simulink model "NInvState"  (R2024b)
settings: Solver=FixedStepDiscrete  StartTime=0.0  StopTime=1  FixedStep=0.001  RelTol=1e-3  EnableMultiTasking=on
settings Model: DataDictionary=Master_Dictionary.sldd  EnableAccessToBaseWorkspace=off  Creator=torni  LastModifiedBy=oxbro
settings SolverCC: AlgebraicLoopSolver=TrustRegion
settings DataIOCC: ReturnWorkspaceOutputs=off
settings OptimizationCC: DefaultParameterBehavior=Inlined  EnhancedBackFolding=on  PassReuseOutputArgsAs=Individual arguments  ZeroExternalMemoryAtStartup=off  ZeroInternalMemoryAtStartup=off  MaxStackSize=512  OptimizeBlockOrder=speed  DifferentSizesBufferReuse=on  OptimizationCustomize=off  EfficientTunableParamExpr=on
settings DebuggingCC: ParameterTunabilityLossMsg=error  UnconnectedInputMsg=warning  UnconnectedOutputMsg=warning  UnconnectedLineMsg=warning  ArithmeticOperatorsInVariantConditions=warning
settings HardwareCC: ProdBitPerPointer=32  ProdBitPerSizeT=32  ProdBitPerPtrDiffT=32  ProdLargestAtomicInteger=Long  ProdLargestAtomicFloat=Double  ProdWordSize=32  ProdLongLongMode=on  ProdHWDeviceType=ARM Compatible->ARM Cortex-M
settings ModelReferenceCC: EnableRefExpFcnMdlSchedulingChecks=on
settings SFSimCC: MATLABDynamicMemAlloc=off  CustomCodeUndefinedFunction=UseInterfaceOnly
settings RTWCC: Description=Embedded Coder  SystemTargetFile=ert.tlc  HardwareBoard=STM32H7xx Based (Single-core)  TemplateMakefile=ert_default_tmf  CustomHeaderCode="#include \"stm32h7xx_ll_tim.h\""  CustomInitializer=LL_TIM_EnableCounter(TIM2);  Toolchain=GNU Tools for ARM Embedded Processors  GPUComputeCapability=3.5
settings CodeAppCC: ForceParamTrailComments=on  IgnoreCustomStorageClasses=off  OperatorAnnotations=on  SimulinkDataObjDesc=on  SFDataObjDesc=on  InsertBlockDesc=on
settings ERTTargetCC: TargetLangStandard=C99 (ISO)  CodeReplacementLibrary=ARM Cortex-M  ExtModeTransport=3  ExtModeStaticAlloc=on  ExtModeStaticAllocSize=2048  ExtModeMexFile=ext_xcp  ExtModeIntrfLevel=Level2 - Open

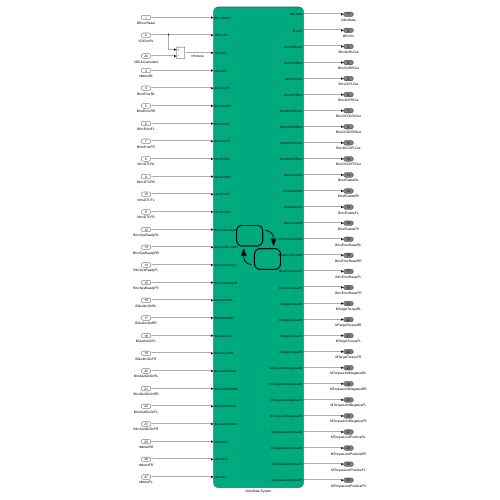
[thumbnail: Simulink's stored preview of the top-level diagram]
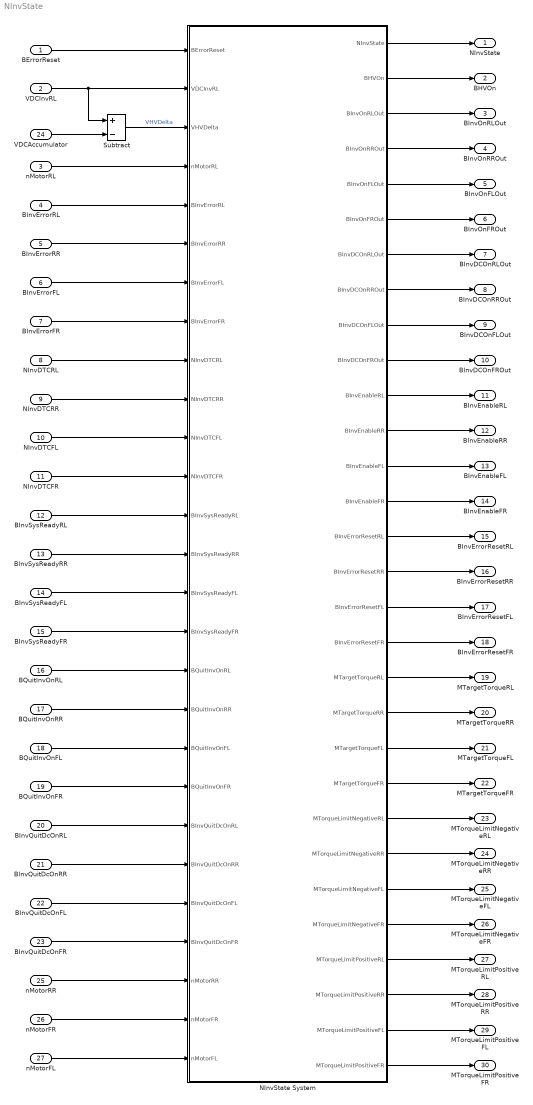
== system NInvState ==
  BErrorReset : Inport  OutDataTypeStr=boolean
  VDCInvRL : Inport  Port=2  OutDataTypeStr=double
  nMotorRL : Inport  Port=3  OutDataTypeStr=double
  BInvErrorRL : Inport  Port=4  OutDataTypeStr=boolean
  BInvErrorRR : Inport  Port=5  OutDataTypeStr=boolean
  BInvErrorFL : Inport  Port=6  OutDataTypeStr=boolean
  BInvErrorFR : Inport  Port=7  OutDataTypeStr=boolean
  NInvDTCRL : Inport  Port=8  OutDataTypeStr=double
  "NInvDTCRR " : Inport  Port=9  OutDataTypeStr=double
  NInvDTCFL : Inport  Port=10  OutDataTypeStr=double
  NInvDTCFR : Inport  Port=11  OutDataTypeStr=double
  BInvSysReadyRL : Inport  Port=12  OutDataTypeStr=boolean
  BInvSysReadyRR : Inport  Port=13  OutDataTypeStr=boolean
  BInvSysReadyFL : Inport  Port=14  OutDataTypeStr=boolean
  BInvSysReadyFR : Inport  Port=15  OutDataTypeStr=boolean
  BQuitInvOnRL : Inport  Port=16  OutDataTypeStr=boolean
  BQuitInvOnRR : Inport  Port=17  OutDataTypeStr=boolean
  BQuitInvOnFL : Inport  Port=18  OutDataTypeStr=boolean
  BQuitInvOnFR : Inport  Port=19  OutDataTypeStr=boolean
  BInvQuitDcOnRL : Inport  Port=20  OutDataTypeStr=boolean
  BInvQuitDcOnRR : Inport  Port=21  OutDataTypeStr=boolean
  BInvQuitDcOnFL : Inport  Port=22  OutDataTypeStr=boolean
  BInvQuitDcOnFR : Inport  Port=23  OutDataTypeStr=boolean
  VDCAccumulator : Inport  Port=24  OutDataTypeStr=double
  nMotorRR : Inport  Port=25  OutDataTypeStr=double
  nMotorFR : Inport  Port=26  OutDataTypeStr=double
  nMotorFL : Inport  Port=27  OutDataTypeStr=double
  NInvState System : Stateflow chart  TreatAsAtomicUnit=on
  Subtract : Sum  Inputs=+-
  NInvState : Outport  OutDataTypeStr=double  VectorParamsAs1DForOutWhenUnconnected=off
  BHVOn : Outport  Port=2  OutDataTypeStr=double  VectorParamsAs1DForOutWhenUnconnected=off
  BInvOnRLOut : Outport  Port=3  OutDataTypeStr=double  VectorParamsAs1DForOutWhenUnconnected=off
  BInvOnRROut : Outport  Port=4  OutDataTypeStr=double  VectorParamsAs1DForOutWhenUnconnected=off
  BInvOnFLOut : Outport  Port=5  OutDataTypeStr=double  VectorParamsAs1DForOutWhenUnconnected=off
  BInvOnFROut : Outport  Port=6  OutDataTypeStr=double  VectorParamsAs1DForOutWhenUnconnected=off
  BInvDCOnRLOut : Outport  Port=7  OutDataTypeStr=double  VectorParamsAs1DForOutWhenUnconnected=off
  BInvDCOnRROut : Outport  Port=8  OutDataTypeStr=double  VectorParamsAs1DForOutWhenUnconnected=off
  BInvDCOnFLOut : Outport  Port=9  OutDataTypeStr=double  VectorParamsAs1DForOutWhenUnconnected=off
  BInvDCOnFROut : Outport  Port=10  OutDataTypeStr=double  VectorParamsAs1DForOutWhenUnconnected=off
  BInvEnableRL : Outport  Port=11  OutDataTypeStr=double  VectorParamsAs1DForOutWhenUnconnected=off
  BInvEnableRR : Outport  Port=12  OutDataTypeStr=double  VectorParamsAs1DForOutWhenUnconnected=off
  BInvEnableFL : Outport  Port=13  OutDataTypeStr=double  VectorParamsAs1DForOutWhenUnconnected=off
  BInvEnableFR : Outport  Port=14  OutDataTypeStr=double  VectorParamsAs1DForOutWhenUnconnected=off
  BInvErrorResetRL : Outport  Port=15  OutDataTypeStr=double  VectorParamsAs1DForOutWhenUnconnected=off
  BInvErrorResetRR : Outport  Port=16  OutDataTypeStr=double  VectorParamsAs1DForOutWhenUnconnected=off
  BInvErrorResetFL : Outport  Port=17  OutDataTypeStr=double  VectorParamsAs1DForOutWhenUnconnected=off
  BInvErrorResetFR : Outport  Port=18  OutDataTypeStr=double  VectorParamsAs1DForOutWhenUnconnected=off
  MTargetTorqueRL : Outport  Port=19  OutDataTypeStr=double  VectorParamsAs1DForOutWhenUnconnected=off
  MTargetTorqueRR : Outport  Port=20  OutDataTypeStr=double  VectorParamsAs1DForOutWhenUnconnected=off
  MTargetTorqueFL : Outport  Port=21  OutDataTypeStr=double  VectorParamsAs1DForOutWhenUnconnected=off
  MTargetTorqueFR : Outport  Port=22  OutDataTypeStr=double  VectorParamsAs1DForOutWhenUnconnected=off
  MTorqueLimitNegativeRL : Outport  Port=23  OutDataTypeStr=double  VectorParamsAs1DForOutWhenUnconnected=off
  MTorqueLimitNegativeRR : Outport  Port=24  OutDataTypeStr=double  VectorParamsAs1DForOutWhenUnconnected=off
  MTorqueLimitNegativeFL : Outport  Port=25  OutDataTypeStr=double  VectorParamsAs1DForOutWhenUnconnected=off
  MTorqueLimitNegativeFR : Outport  Port=26  OutDataTypeStr=double  VectorParamsAs1DForOutWhenUnconnected=off
  MTorqueLimitPositiveRL : Outport  Port=27  OutDataTypeStr=double  VectorParamsAs1DForOutWhenUnconnected=off
  MTorqueLimitPositiveRR : Outport  Port=28  OutDataTypeStr=double  VectorParamsAs1DForOutWhenUnconnected=off
  MTorqueLimitPositiveFL : Outport  Port=29  OutDataTypeStr=double  VectorParamsAs1DForOutWhenUnconnected=off
  MTorqueLimitPositiveFR : Outport  Port=30  OutDataTypeStr=double  VectorParamsAs1DForOutWhenUnconnected=off
  wires:
  BErrorReset/1 -> NInvState System/1(BErrorReset)
  VDCInvRL/1 -> Subtract/1, NInvState System/2(VDCInvRL)
  nMotorRL/1 -> NInvState System/4(nMotorRL)
  BInvErrorRL/1 -> NInvState System/5(BInvErrorRL)
  BInvErrorRR/1 -> NInvState System/6(BInvErrorRR)
  BInvErrorFL/1 -> NInvState System/7(BInvErrorFL)
  BInvErrorFR/1 -> NInvState System/8(BInvErrorFR)
  NInvDTCRL/1 -> NInvState System/9(NInvDTCRL)
  "NInvDTCRR "/1 -> NInvState System/10(NInvDTCRR)
  NInvDTCFL/1 -> NInvState System/11(NInvDTCFL)
  NInvDTCFR/1 -> NInvState System/12(NInvDTCFR)
  BInvSysReadyRL/1 -> NInvState System/13(BInvSysReadyRL)
  BInvSysReadyRR/1 -> NInvState System/14(BInvSysReadyRR)
  BInvSysReadyFL/1 -> NInvState System/15(BInvSysReadyFL)
  BInvSysReadyFR/1 -> NInvState System/16(BInvSysReadyFR)
  BQuitInvOnRL/1 -> NInvState System/17(BQuitInvOnRL)
  BQuitInvOnRR/1 -> NInvState System/18(BQuitInvOnRR)
  BQuitInvOnFL/1 -> NInvState System/19(BQuitInvOnFL)
  BQuitInvOnFR/1 -> NInvState System/20(BQuitInvOnFR)
  BInvQuitDcOnRL/1 -> NInvState System/21(BInvQuitDcOnRL)
  BInvQuitDcOnFL/1 -> NInvState System/23(BInvQuitDcOnFL)
  BInvQuitDcOnRR/1 -> NInvState System/22(BInvQuitDcOnRR)
  BInvQuitDcOnFR/1 -> NInvState System/24(BInvQuitDcOnFR)
  VDCAccumulator/1 -> Subtract/2
  Subtract/1 -> NInvState System/3(VHVDelta)  "VHVDelta"
  NInvState System/2(BHVOn) -> BHVOn/1
  NInvState System/1(NInvState) -> NInvState/1
  NInvState System/3(BInvOnRLOut) -> BInvOnRLOut/1
  NInvState System/4(BInvOnRROut) -> BInvOnRROut/1
  NInvState System/5(BInvOnFLOut) -> BInvOnFLOut/1
  NInvState System/6(BInvOnFROut) -> BInvOnFROut/1
  NInvState System/7(BInvDCOnRLOut) -> BInvDCOnRLOut/1
  NInvState System/8(BInvDCOnRROut) -> BInvDCOnRROut/1
  NInvState System/9(BInvDCOnFLOut) -> BInvDCOnFLOut/1
  NInvState System/10(BInvDCOnFROut) -> BInvDCOnFROut/1
  NInvState System/11(BInvEnableRL) -> BInvEnableRL/1
  NInvState System/12(BInvEnableRR) -> BInvEnableRR/1
  NInvState System/13(BInvEnableFL) -> BInvEnableFL/1
  NInvState System/14(BInvEnableFR) -> BInvEnableFR/1
  NInvState System/15(BInvErrorResetRL) -> BInvErrorResetRL/1
  NInvState System/16(BInvErrorResetRR) -> BInvErrorResetRR/1
  NInvState System/17(BInvErrorResetFL) -> BInvErrorResetFL/1
  NInvState System/18(BInvErrorResetFR) -> BInvErrorResetFR/1
  NInvState System/19(MTargetTorqueRL) -> MTargetTorqueRL/1
  NInvState System/20(MTargetTorqueRR) -> MTargetTorqueRR/1
  NInvState System/21(MTargetTorqueFL) -> MTargetTorqueFL/1
  NInvState System/22(MTargetTorqueFR) -> MTargetTorqueFR/1
  NInvState System/23(MTorqueLimitNegativeRL) -> MTorqueLimitNegativeRL/1
  NInvState System/24(MTorqueLimitNegativeRR) -> MTorqueLimitNegativeRR/1
  NInvState System/25(MTorqueLimitNegativeFL) -> MTorqueLimitNegativeFL/1
  NInvState System/26(MTorqueLimitNegativeFR) -> MTorqueLimitNegativeFR/1
  NInvState System/27(MTorqueLimitPositiveRL) -> MTorqueLimitPositiveRL/1
  NInvState System/28(MTorqueLimitPositiveRR) -> MTorqueLimitPositiveRR/1
  NInvState System/29(MTorqueLimitPositiveFL) -> MTorqueLimitPositiveFL/1
  NInvState System/30(MTorqueLimitPositiveFR) -> MTorqueLimitPositiveFR/1
  nMotorRR/1 -> NInvState System/25(nMotorRR)
  nMotorFR/1 -> NInvState System/26(nMotorFR)
  nMotorFL/1 -> NInvState System/27(nMotorFL)

== stateflow chart NInvState/NInvState System ==
  state Inv_State_Idle
    entry:
    NInvState=0;
  state Inverter_DCOFF
    entry:
    BInvDCOnFLOut = 0
    BInvDCOnFROut = 0
    BInvDCOnRLOut = 0
    BInvDCOnRROut = 0
  state Inv_Error_Checks
    state Inv_LV_Check2
      entry:
      NInvState=2
      BInvErrorResetRR=0;
      BInvErrorResetRL=0;
      BInvErrorResetFR=0;
      BInvErrorResetFL=0;
    state Inv_LV_Check1
      entry:
      BInvErrorResetRR=1;
      BInvErrorResetRL=1;
      BInvErrorResetFR=1;
      BInvErrorResetFL=1;
    state Inv_LV_OK
      entry:
      NInvState=3;
    state Inv_LV_Check
      entry:
      NInvState=1;
      BInvErrorResetRR=0;
      BInvErrorResetRL=0;
      BInvErrorResetFR=0;
      BInvErrorResetFL=0;
    Inv_LV_Check1 -> Inv_LV_Check2 : after(100, tick)
        | [BInvErrorFL==0&&...
        | BInvErrorFR==0&&...
        | BInvErrorRR==0&&...
        | BInvErrorRL==0]
    (default) -> Inv_LV_Check
    Inv_LV_Check2 -> Inv_LV_Check [order 1] : [BInvErrorRR==1 ||...
        | BInvErrorRL==1 ||...
        | BInvErrorFR==1 ||...
        | BInvErrorFL==1]
    Inv_LV_Check2 -> Inv_LV_OK [order 2] : [BInvErrorRR==0 &&...
        | BInvErrorRL==0 &&...
        | BInvErrorFR==0 &&...
        | BInvErrorFL==0 &&...
        | BInvSysReadyRL==1 &&...
        | BInvSysReadyRR==1 &&...
        | BInvSysReadyFL==1 &&...
        | BInvSysReadyFR==1]
    Inv_LV_Check -> Inv_LV_Check1 : after(100,tick)
    Inv_LV_OK -> Inv_LV_Check : [BErrorReset==1 && nMotorRL<500]
  state Inv_OK
    entry:
    NInvState=92
  state Encoder_Reset_RL
    state Encoder_Error_RL
      entry:
      NInvState=404
      state PBX_SENSORS_ini
        entry:
        BInvErrorResetRL=0;
      state Error_On
        entry:
        BInvErrorResetRL=1;
      state Error_off
        entry:
        BInvErrorResetRL=0;
      (default) -> Encoder_Reset_RL.Encoder_Error_RL.PBX_SENSORS_ini
      Encoder_Reset_RL.Encoder_Error_RL.PBX_SENSORS_ini -> Encoder_Reset_RL.Encoder_Error_RL.Error_On : after(50, tick)
      Encoder_Reset_RL.Encoder_Error_RL.Error_off -> Encoder_Reset_RL.Encoder_Error_RL.PBX_SENSORS_ini [order 2] : [BInvErrorRL ==1]
      Encoder_Reset_RL.Encoder_Error_RL.Error_On -> Encoder_Reset_RL.Encoder_Error_RL.Error_off : after(100, tick)
          | [BInvErrorRL ==0]
    state Inverter_HV_Checks3
      exit:
      BHVOn=1
      state Inverter_IN
        entry:
        NInvState = 22
        BInvDCOnRLOut = 1
      state Inv_Error_Check_2
        BInvErrorResetRL = 0
      state Inv_Error_Reset
        entry:
        BInvErrorResetRL=1
        BInvDCOnRLOut=0
        BInvEnableRL = 0
        BInvOnRLOut = 0
      state START_UP
        entry:
        NInvState = 23
        MTargetTorqueRL=0
        MTorqueLimitNegativeRL = 0
        MTorqueLimitPositiveRL = 0
        BInvEnableRL = 1
      state Inv_Error_Check_1
        entry:
        NInvState = 00
        MTorqueLimitNegativeRL = 0
        MTorqueLimitPositiveRL = 0
      state Inverter_ON
        entry:
        NInvState = 24
        BInvOnRLOut = 1
      state TorqueReq_Ready
        entry:
        NInvState = 25
        MTorqueLimitNegativeRL = -204.1
        MTorqueLimitPositiveRL = 214.2
      (default) -> Encoder_Reset_RL.Inverter_HV_Checks3.Inverter_IN
      (junction 784) -> Encoder_Reset_RL.Inverter_HV_Checks3.Inverter_IN [order 1] : [BInvErrorRL==0]
      Encoder_Reset_RL.Inverter_HV_Checks3.Inv_Error_Check_2 -> (junction 784) : after(500,tick)
      (junction 784) -> Encoder_Reset_RL.Inverter_HV_Checks3.Inv_Error_Check_1 [order 2] : [BInvErrorRL==1]
      Encoder_Reset_RL.Inverter_HV_Checks3.Inv_Error_Reset -> Encoder_Reset_RL.Inverter_HV_Checks3.Inv_Error_Check_2 : after(500,tick)
      Encoder_Reset_RL.Inverter_HV_Checks3.Inverter_IN -> Encoder_Reset_RL.Inverter_HV_Checks3.START_UP : [BInvQuitDcOnRL==1]
      Encoder_Reset_RL.Inverter_HV_Checks3.START_UP -> Encoder_Reset_RL.Inverter_HV_Checks3.Inverter_ON : after(100,tick)
      Encoder_Reset_RL.Inverter_HV_Checks3.Inv_Error_Check_1 -> Encoder_Reset_RL.Inverter_HV_Checks3.Inv_Error_Reset : after(500,tick)
      Encoder_Reset_RL.Inverter_HV_Checks3.Inverter_ON -> Encoder_Reset_RL.Inverter_HV_Checks3.TorqueReq_Ready [order 1] : [BQuitInvOnRL == 1]
      Encoder_Reset_RL.Inverter_HV_Checks3.Inverter_ON -> Encoder_Reset_RL.Inverter_HV_Checks3.Inv_Error_Check_1 [order 2] : [BInvErrorRL==1]
      Encoder_Reset_RL.Inverter_HV_Checks3.TorqueReq_Ready -> Encoder_Reset_RL.Inverter_HV_Checks3.Inv_Error_Check_1 [order 1] : [BInvErrorRL==1]
    state Encoder_OK
      entry:
      NInvState = 26
    (default) -> Encoder_Error_RL
    Encoder_Reset_RL.Encoder_Error_RL.Error_off -> Encoder_Reset_RL.Inverter_HV_Checks3 [order 1] : [BInvSysReadyRL==1]
    Encoder_Reset_RL.Inverter_HV_Checks3.TorqueReq_Ready -> Encoder_Reset_RL.Encoder_OK [order 2] : [BInvErrorRL==0]
  state Encoder_Reset_RR
    state Encoder_Error_RR
      entry:
      NInvState = 404
      state PBX_SENSORS_ini
        entry:
        BInvErrorResetRR=0;
      state Error_On
        entry:
        BInvErrorResetRR=1;
      state Error_off
        entry:
        BInvErrorResetRR=0;
      (default) -> Encoder_Reset_RR.Encoder_Error_RR.PBX_SENSORS_ini
      Encoder_Reset_RR.Encoder_Error_RR.PBX_SENSORS_ini -> Encoder_Reset_RR.Encoder_Error_RR.Error_On : after(50, tick)
      Encoder_Reset_RR.Encoder_Error_RR.Error_off -> Encoder_Reset_RR.Encoder_Error_RR.PBX_SENSORS_ini [order 2] : [BInvErrorRR ==1]
      Encoder_Reset_RR.Encoder_Error_RR.Error_On -> Encoder_Reset_RR.Encoder_Error_RR.Error_off : after(100, tick)
          | [BInvErrorRR ==0]
    state Inverter_HV_CheckRR
      exit:
      BHVOn=1
      state Inverter_IN
        entry:
        NInvState = 27
        BInvDCOnRROut = 1
      state Inv_Error_Check_2
        BInvErrorResetRR = 0
      state Inv_Error_Reset
        entry:
        BInvErrorResetRR=1
        BInvDCOnRROut=0
        BInvEnableRR = 0
        BInvOnRROut = 0
      state START_UP
        entry:
        NInvState = 28
        MTargetTorqueRR=0
        MTorqueLimitNegativeRR = 0
        MTorqueLimitPositiveRR = 0
        BInvEnableRR = 1
      state Inv_Error_Check_1
        entry:
        MTorqueLimitNegativeRR = 0
        MTorqueLimitPositiveRR = 0
      state Inverter_ON
        entry:
        NInvState = 29
        BInvOnRROut = 1
      state TorqueReq_Ready
        entry:
        NInvState = 30
        MTorqueLimitNegativeRR = -204.1
        MTorqueLimitPositiveRR = 214.2
      (default) -> Encoder_Reset_RR.Inverter_HV_CheckRR.Inverter_IN
      (junction 861) -> Encoder_Reset_RR.Inverter_HV_CheckRR.Inverter_IN [order 1] : [BInvErrorRR==0]
      Encoder_Reset_RR.Inverter_HV_CheckRR.Inv_Error_Check_2 -> (junction 861) : after(500,tick)
      (junction 861) -> Encoder_Reset_RR.Inverter_HV_CheckRR.Inv_Error_Check_1 [order 2] : [BInvErrorRR==1]
      Encoder_Reset_RR.Inverter_HV_CheckRR.Inv_Error_Reset -> Encoder_Reset_RR.Inverter_HV_CheckRR.Inv_Error_Check_2 : after(500,tick)
      Encoder_Reset_RR.Inverter_HV_CheckRR.Inverter_IN -> Encoder_Reset_RR.Inverter_HV_CheckRR.START_UP : [BInvQuitDcOnRR==1]
      Encoder_Reset_RR.Inverter_HV_CheckRR.START_UP -> Encoder_Reset_RR.Inverter_HV_CheckRR.Inverter_ON : after(100,tick)
      Encoder_Reset_RR.Inverter_HV_CheckRR.Inv_Error_Check_1 -> Encoder_Reset_RR.Inverter_HV_CheckRR.Inv_Error_Reset : after(500,tick)
      Encoder_Reset_RR.Inverter_HV_CheckRR.Inverter_ON -> Encoder_Reset_RR.Inverter_HV_CheckRR.TorqueReq_Ready [order 1] : [BQuitInvOnRR == 1]
      Encoder_Reset_RR.Inverter_HV_CheckRR.Inverter_ON -> Encoder_Reset_RR.Inverter_HV_CheckRR.Inv_Error_Check_1 [order 2] : [BInvErrorRR==1]
      Encoder_Reset_RR.Inverter_HV_CheckRR.TorqueReq_Ready -> Encoder_Reset_RR.Inverter_HV_CheckRR.Inv_Error_Check_1 [order 1] : [BInvErrorRR==1]
    state Encoder_OK
      entry:
      NInvState = 31
    (default) -> Encoder_Error_RR
    Encoder_Reset_RR.Encoder_Error_RR.Error_off -> Encoder_Reset_RR.Inverter_HV_CheckRR [order 1] : [BInvSysReadyRR==1]
    Encoder_Reset_RR.Inverter_HV_CheckRR.TorqueReq_Ready -> Encoder_Reset_RR.Encoder_OK [order 2] : [BInvErrorRR==0]
  state Encoder_Reset_FL
    state Encoder_Error_FL
      entry:
      NInvState = 404
      state Error_On
        entry:
        BInvErrorResetFL=1;
      state PBX_SENSORS_ini
        entry:
        BInvErrorResetFL=0;
      state Error_off
        entry:
        BInvErrorResetFL=0;
      (default) -> Encoder_Reset_FL.Encoder_Error_FL.PBX_SENSORS_ini
      Encoder_Reset_FL.Encoder_Error_FL.PBX_SENSORS_ini -> Encoder_Reset_FL.Encoder_Error_FL.Error_On : after(50, tick)
      Encoder_Reset_FL.Encoder_Error_FL.Error_off -> Encoder_Reset_FL.Encoder_Error_FL.PBX_SENSORS_ini [order 2] : [BInvErrorFL ==1]
      Encoder_Reset_FL.Encoder_Error_FL.Error_On -> Encoder_Reset_FL.Encoder_Error_FL.Error_off : after(100, tick)
          | [BInvErrorFL ==0]
    state Inverter_HV_Checks2
      exit:
      BHVOn=1
      state Inverter_IN
        entry:
        NInvState = 32
        BInvDCOnFLOut = 1
      state Inv_Error_Check_2
        BInvErrorResetFL = 0
      state Inv_Error_Reset
        entry:
        BInvErrorResetFL=1
        BInvDCOnFLOut=0
        BInvEnableFL = 0
        BInvOnFLOut = 0
      state START_UP
        entry:
        NInvState = 33
        MTargetTorqueFL=0
        MTorqueLimitNegativeFL = 0
        MTorqueLimitPositiveFL = 0
        BInvEnableFL = 1
      state Inv_Error_Check_1
        entry:
        MTorqueLimitNegativeFL = 0
        MTorqueLimitPositiveFL = 0
      state Inverter_ON
        entry:
        NInvState = 34
        BInvOnFLOut = 1
      state TorqueReq_Ready
        entry:
        NInvState = 35
        MTorqueLimitNegativeFL = -204.1
        MTorqueLimitPositiveFL = 214.2
      (default) -> Encoder_Reset_FL.Inverter_HV_Checks2.Inverter_IN
      (junction 751) -> Encoder_Reset_FL.Inverter_HV_Checks2.Inverter_IN [order 1] : [BInvErrorFL==0]
      Encoder_Reset_FL.Inverter_HV_Checks2.Inv_Error_Check_2 -> (junction 751) : after(500,tick)
      (junction 751) -> Encoder_Reset_FL.Inverter_HV_Checks2.Inv_Error_Check_1 [order 2] : [BInvErrorFL==1]
      Encoder_Reset_FL.Inverter_HV_Checks2.Inv_Error_Reset -> Encoder_Reset_FL.Inverter_HV_Checks2.Inv_Error_Check_2 : after(500,tick)
      Encoder_Reset_FL.Inverter_HV_Checks2.Inverter_IN -> Encoder_Reset_FL.Inverter_HV_Checks2.START_UP : [BInvQuitDcOnFL==1]
      Encoder_Reset_FL.Inverter_HV_Checks2.START_UP -> Encoder_Reset_FL.Inverter_HV_Checks2.Inverter_ON : after(100,tick)
      Encoder_Reset_FL.Inverter_HV_Checks2.Inv_Error_Check_1 -> Encoder_Reset_FL.Inverter_HV_Checks2.Inv_Error_Reset : after(500,tick)
      Encoder_Reset_FL.Inverter_HV_Checks2.Inverter_ON -> Encoder_Reset_FL.Inverter_HV_Checks2.TorqueReq_Ready [order 1] : [BQuitInvOnFL == 1]
      Encoder_Reset_FL.Inverter_HV_Checks2.Inverter_ON -> Encoder_Reset_FL.Inverter_HV_Checks2.Inv_Error_Check_1 [order 2] : [BInvErrorFL==1]
      Encoder_Reset_FL.Inverter_HV_Checks2.TorqueReq_Ready -> Encoder_Reset_FL.Inverter_HV_Checks2.Inv_Error_Check_1 [order 1] : [BInvErrorFL==1]
    state Encoder_OK
      entry:
      NInvState = 36
    (default) -> Encoder_Error_FL
    Encoder_Reset_FL.Encoder_Error_FL.Error_off -> Inverter_HV_Checks2 [order 1] : [BInvSysReadyFL==1]
    Encoder_Reset_FL.Inverter_HV_Checks2.TorqueReq_Ready -> Encoder_Reset_FL.Encoder_OK [order 2] : [BInvErrorFL==0]
  state Inverter_HV_Checks
    state Inverter_HV_CheckFR
      exit:
      BHVOn=1;
      NInvState = 4
      state Inverter_IN
        entry:
        NInvState = 5
        BInvDCOnFROut = 1
      state Inv_Error_Check_2
        BInvErrorResetFR = 0
      state Inv_Error_Reset
        entry:
        BInvErrorResetFR=1
        BInvDCOnFROut=0
        BInvEnableFR = 0
        BInvOnFROut = 0
      state START_UP
        entry:
        NInvState = 6
        MTargetTorqueFR=0
        MTorqueLimitNegativeFR = 0
        MTorqueLimitPositiveFR = 0
        BInvEnableFR = 1
      state Inv_Error_Check_1
        entry:
        MTorqueLimitNegativeFR = 0
        MTorqueLimitPositiveFR = 0
      state Inverter_ON
        entry:
        NInvState = 7
        BInvOnFROut = 1
      state TorqueReq_Ready
        entry:
        NInvState = 8
        MTorqueLimitNegativeFR = -204.1
        MTorqueLimitPositiveFR = 214.2
      (default) -> Inverter_HV_Checks.Inverter_HV_CheckFR.Inverter_IN
      (junction 1179) -> Inverter_HV_Checks.Inverter_HV_CheckFR.Inverter_IN [order 1] : [BInvErrorFR==0]
      Inverter_HV_Checks.Inverter_HV_CheckFR.Inv_Error_Check_2 -> (junction 1179) : after(500,tick)
      (junction 1179) -> Inverter_HV_Checks.Inverter_HV_CheckFR.Inv_Error_Check_1 [order 2] : [BInvErrorFR==1]
      Inverter_HV_Checks.Inverter_HV_CheckFR.Inverter_IN -> Inverter_HV_Checks.Inverter_HV_CheckFR.Inv_Error_Reset [order 2] : after(500,tick)[BInvErrorFR==1]
      Inverter_HV_Checks.Inverter_HV_CheckFR.Inv_Error_Reset -> Inverter_HV_Checks.Inverter_HV_CheckFR.Inv_Error_Check_2 : after(500,tick)
      Inverter_HV_Checks.Inverter_HV_CheckFR.Inverter_IN -> Inverter_HV_Checks.Inverter_HV_CheckFR.START_UP [order 1] : [BInvQuitDcOnFR==1]
      Inverter_HV_Checks.Inverter_HV_CheckFR.START_UP -> Inverter_HV_Checks.Inverter_HV_CheckFR.Inverter_ON : after(100,tick)
      Inverter_HV_Checks.Inverter_HV_CheckFR.Inv_Error_Check_1 -> Inverter_HV_Checks.Inverter_HV_CheckFR.Inv_Error_Reset : after(500,tick)
      Inverter_HV_Checks.Inverter_HV_CheckFR.Inverter_ON -> Inverter_HV_Checks.Inverter_HV_CheckFR.TorqueReq_Ready [order 1] : [BQuitInvOnFR == 1]
      Inverter_HV_Checks.Inverter_HV_CheckFR.Inverter_ON -> Inverter_HV_Checks.Inverter_HV_CheckFR.Inv_Error_Check_1 [order 2] : [BInvErrorFR==1]
      Inverter_HV_Checks.Inverter_HV_CheckFR.TorqueReq_Ready -> Inverter_HV_Checks.Inverter_HV_CheckFR.Inv_Error_Check_1 [order 2] : [BInvErrorFR==1]
    state Inv_HV_Check
    note: FRONT RIGHT INVERTER
    state Inverter_HV_CheckRR
      exit:
      BHVOn=1
      state Inverter_IN
        entry:
        NInvState = 9;
        BInvDCOnRROut = 1
      state Inv_Error_Check_2
        BInvErrorResetRR = 0
      state Inv_Error_Reset
        entry:
        BInvErrorResetRR=1
        BInvDCOnRROut=0
        BInvEnableRR = 0
        BInvOnRROut = 0
      state START_UP
        entry:
        NInvState = 10
        MTargetTorqueRR=0
        MTorqueLimitNegativeRR = 0
        MTorqueLimitPositiveRR = 0
        BInvEnableRR = 1
      state Inv_Error_Check_1
        entry:
        MTorqueLimitNegativeRR = 0
        MTorqueLimitPositiveRR = 0
      state Inverter_ON
        entry:
        NInvState = 11
        BInvOnRROut = 1
      state TorqueReq_Ready
        entry:
        NInvState = 12
        MTorqueLimitNegativeRR = -204.1
        MTorqueLimitPositiveRR = 214.2
      (default) -> Inverter_HV_Checks.Inverter_HV_CheckRR.Inverter_IN
      (junction 1201) -> Inverter_HV_Checks.Inverter_HV_CheckRR.Inverter_IN [order 1] : [BInvErrorRR==0]
      Inverter_HV_Checks.Inverter_HV_CheckRR.Inv_Error_Check_2 -> (junction 1201) : after(500,tick)
      (junction 1201) -> Inverter_HV_Checks.Inverter_HV_CheckRR.Inv_Error_Check_1 [order 2] : [BInvErrorRR==1]
      Inverter_HV_Checks.Inverter_HV_CheckRR.Inverter_IN -> Inverter_HV_Checks.Inverter_HV_CheckRR.Inv_Error_Reset [order 2] : after(500,tick)[BInvErrorRR==1]
      Inverter_HV_Checks.Inverter_HV_CheckRR.Inv_Error_Reset -> Inverter_HV_Checks.Inverter_HV_CheckRR.Inv_Error_Check_2 : after(500,tick)
      Inverter_HV_Checks.Inverter_HV_CheckRR.Inverter_IN -> Inverter_HV_Checks.Inverter_HV_CheckRR.START_UP [order 1] : [BInvQuitDcOnRR==1]
      Inverter_HV_Checks.Inverter_HV_CheckRR.START_UP -> Inverter_HV_Checks.Inverter_HV_CheckRR.Inverter_ON : after(100,tick)
      Inverter_HV_Checks.Inverter_HV_CheckRR.Inv_Error_Check_1 -> Inverter_HV_Checks.Inverter_HV_CheckRR.Inv_Error_Reset : after(500,tick)
      Inverter_HV_Checks.Inverter_HV_CheckRR.Inverter_ON -> Inverter_HV_Checks.Inverter_HV_CheckRR.TorqueReq_Ready [order 1] : [BQuitInvOnRR == 1]
      Inverter_HV_Checks.Inverter_HV_CheckRR.Inverter_ON -> Inverter_HV_Checks.Inverter_HV_CheckRR.Inv_Error_Check_1 [order 2] : [BInvErrorRR==1]
      Inverter_HV_Checks.Inverter_HV_CheckRR.TorqueReq_Ready -> Inverter_HV_Checks.Inverter_HV_CheckRR.Inv_Error_Check_1 [order 2] : [BInvErrorRR==1]
    note: REAR RIGHT INVERTER
    state Inverter_HV_ChecksFL
      exit:
      BHVOn=1
      state Inverter_IN
        entry:
        NInvState = 13
        BInvDCOnFLOut = 1
      state Inv_Error_Check_2
        BInvErrorResetFL = 0
      state Inv_Error_Reset
        entry:
        BInvErrorResetFL=1
        BInvDCOnFLOut=0
        BInvEnableFL = 0
        BInvOnFLOut = 0
      state START_UP
        entry:
        NInvState = 14
        MTargetTorqueFL=0
        MTorqueLimitNegativeFL = 0
        MTorqueLimitPositiveFL = 0
        BInvEnableFL = 1
      state Inv_Error_Check_1
        entry:
        MTorqueLimitNegativeFL = 0
        MTorqueLimitPositiveFL = 0
      state Inverter_ON
        entry:
        NInvState = 15
        BInvOnFLOut = 1
      state TorqueReq_Ready
        entry:
        NInvState = 16
        MTorqueLimitNegativeFL = -204.1
        MTorqueLimitPositiveFL = 214.2
      (default) -> Inverter_HV_Checks.Inverter_HV_ChecksFL.Inverter_IN
      (junction 1222) -> Inverter_HV_Checks.Inverter_HV_ChecksFL.Inverter_IN [order 1] : [BInvErrorFL==0]
      Inverter_HV_Checks.Inverter_HV_ChecksFL.Inv_Error_Check_2 -> (junction 1222) : after(500,tick)
      (junction 1222) -> Inverter_HV_Checks.Inverter_HV_ChecksFL.Inv_Error_Check_1 [order 2] : [BInvErrorFL==1]
      Inverter_HV_Checks.Inverter_HV_ChecksFL.Inverter_IN -> Inverter_HV_Checks.Inverter_HV_ChecksFL.Inv_Error_Reset [order 2] : after(500,tick)[BInvErrorFL==1]
      Inverter_HV_Checks.Inverter_HV_ChecksFL.Inv_Error_Reset -> Inverter_HV_Checks.Inverter_HV_ChecksFL.Inv_Error_Check_2 : after(500,tick)
      Inverter_HV_Checks.Inverter_HV_ChecksFL.Inverter_IN -> Inverter_HV_Checks.Inverter_HV_ChecksFL.START_UP [order 1] : [BInvQuitDcOnFL==1]
      Inverter_HV_Checks.Inverter_HV_ChecksFL.START_UP -> Inverter_HV_Checks.Inverter_HV_ChecksFL.Inverter_ON : after(100,tick)
      Inverter_HV_Checks.Inverter_HV_ChecksFL.Inv_Error_Check_1 -> Inverter_HV_Checks.Inverter_HV_ChecksFL.Inv_Error_Reset : after(500,tick)
      Inverter_HV_Checks.Inverter_HV_ChecksFL.Inverter_ON -> Inverter_HV_Checks.Inverter_HV_ChecksFL.TorqueReq_Ready [order 1] : [BQuitInvOnFL == 1]
      Inverter_HV_Checks.Inverter_HV_ChecksFL.Inverter_ON -> Inverter_HV_Checks.Inverter_HV_ChecksFL.Inv_Error_Check_1 [order 2] : [BInvErrorFL==1]
      Inverter_HV_Checks.Inverter_HV_ChecksFL.TorqueReq_Ready -> Inverter_HV_Checks.Inverter_HV_ChecksFL.Inv_Error_Check_1 [order 2] : [BInvErrorFL==1]
    note: FRONT LEFT INVERTER
    state Inverter_HV_ChecksRL
      exit:
      BHVOn=1
      state Inverter_IN
        entry:
        NInvState = 17
        BInvDCOnRLOut = 1
      state Inv_Error_Check_2
        BInvErrorResetRL = 0
      state Inv_Error_Reset
        entry:
        BInvErrorResetRL=1
        BInvDCOnRLOut=0
        BInvEnableRL = 0
        BInvOnRLOut = 0
      state START_UP
        entry:
        NInvState = 18
        MTargetTorqueRL=0
        MTorqueLimitNegativeRL = 0
        MTorqueLimitPositiveRL = 0
        BInvEnableRL = 1
      state Inv_Error_Check_1
        entry:
        MTorqueLimitNegativeRL = 0
        MTorqueLimitPositiveRL = 0
      state Inverter_ON
        entry:
        NInvState = 19
        BInvOnRLOut = 1
      state TorqueReq_Ready
        entry:
        NInvState = 20
        MTorqueLimitNegativeRL = -204.1
        MTorqueLimitPositiveRL = 214.2
      (default) -> Inverter_HV_Checks.Inverter_HV_ChecksRL.Inverter_IN
      (junction 1243) -> Inverter_HV_Checks.Inverter_HV_ChecksRL.Inverter_IN [order 1] : [BInvErrorRL==0]
      Inverter_HV_Checks.Inverter_HV_ChecksRL.Inv_Error_Check_2 -> (junction 1243) : after(500,tick)
      (junction 1243) -> Inverter_HV_Checks.Inverter_HV_ChecksRL.Inv_Error_Check_1 [order 2] : [BInvErrorRL==1]
      Inverter_HV_Checks.Inverter_HV_ChecksRL.Inverter_IN -> Inverter_HV_Checks.Inverter_HV_ChecksRL.Inv_Error_Reset [order 2] : after(500,tick)[BInvErrorRL==1]
      Inverter_HV_Checks.Inverter_HV_ChecksRL.Inv_Error_Reset -> Inverter_HV_Checks.Inverter_HV_ChecksRL.Inv_Error_Check_2 : after(500,tick)
      Inverter_HV_Checks.Inverter_HV_ChecksRL.Inverter_IN -> Inverter_HV_Checks.Inverter_HV_ChecksRL.START_UP [order 1] : [BInvQuitDcOnRL==1]
      Inverter_HV_Checks.Inverter_HV_ChecksRL.START_UP -> Inverter_HV_Checks.Inverter_HV_ChecksRL.Inverter_ON : after(100,tick)
      Inverter_HV_Checks.Inverter_HV_ChecksRL.Inv_Error_Check_1 -> Inverter_HV_Checks.Inverter_HV_ChecksRL.Inv_Error_Reset : after(500,tick)
      Inverter_HV_Checks.Inverter_HV_ChecksRL.Inverter_ON -> Inverter_HV_Checks.Inverter_HV_ChecksRL.TorqueReq_Ready [order 1] : [BQuitInvOnRL == 1]
      Inverter_HV_Checks.Inverter_HV_ChecksRL.Inverter_ON -> Inverter_HV_Checks.Inverter_HV_ChecksRL.Inv_Error_Check_1 [order 2] : [BInvErrorRL==1]
      Inverter_HV_Checks.Inverter_HV_ChecksRL.TorqueReq_Ready -> Inverter_HV_Checks.Inverter_HV_ChecksRL.Inv_Error_Check_1 [order 1] : [BInvErrorRL==1]
    note: REAR LEFT INVERTER
    state Inv_OK
      entry:
      NInvState = 21;
    (default) -> Inv_HV_Check
    Inv_HV_Check -> Inverter_HV_CheckFR : [NInvState==3]
    Inverter_HV_Checks.Inverter_HV_CheckFR.TorqueReq_Ready -> Inverter_HV_Checks.Inverter_HV_CheckRR [order 1] : after(500,tick)[BInvErrorFR==0]
    Inverter_HV_Checks.Inverter_HV_CheckRR.TorqueReq_Ready -> Inverter_HV_ChecksFL [order 1] : after(500,tick)[BInvErrorRR==0]
    Inverter_HV_Checks.Inverter_HV_ChecksFL.TorqueReq_Ready -> Inverter_HV_ChecksRL [order 1] : after(500,tick)[BInvErrorFL==0]
    Inverter_HV_Checks.Inverter_HV_ChecksRL.TorqueReq_Ready -> Inverter_HV_Checks.Inv_OK [order 2] : [BInvErrorRL==0]
  state Encoder_Reset_FR
    state Encoder_Error_FR
      entry:
      NInvState = 404
      state PBX_SENSORS_ini
        entry:
        BInvErrorResetFR=0;
      state Error_On
        entry:
        BInvErrorResetFR=1;
      state Error_off
        entry:
        BInvErrorResetFR=0;
      (default) -> Encoder_Reset_FR.Encoder_Error_FR.PBX_SENSORS_ini
      Encoder_Reset_FR.Encoder_Error_FR.PBX_SENSORS_ini -> Encoder_Reset_FR.Encoder_Error_FR.Error_On : after(50, tick)
      Encoder_Reset_FR.Encoder_Error_FR.Error_off -> Encoder_Reset_FR.Encoder_Error_FR.PBX_SENSORS_ini [order 2] : [BInvErrorFR ==1]
      Encoder_Reset_FR.Encoder_Error_FR.Error_On -> Encoder_Reset_FR.Encoder_Error_FR.Error_off : after(100, tick)
          | [BInvErrorFR ==0]
    state Inverter_HV_Checks3
      exit:
      BHVOn=1
      state Inverter_IN
        entry:
        NInvState = 37
        BInvDCOnFROut = 1
      state Inv_Error_Check_2
        BInvErrorResetFR = 0
      state Inv_Error_Reset
        entry:
        BInvErrorResetFR=1
        BInvDCOnFROut=0
        BInvEnableFR = 0
        BInvOnFROut = 0
      state START_UP
        entry:
        NInvState = 38
        MTargetTorqueFR=0
        MTorqueLimitNegativeFR = 0
        MTorqueLimitPositiveFR = 0
        BInvEnableFR = 1
      state Inv_Error_Check_1
        entry:
        MTorqueLimitNegativeFR = 0
        MTorqueLimitPositiveFR = 0
      state Inverter_ON
        entry:
        NInvState = 39
        BInvOnFROut = 1
      state TorqueReq_Ready
        entry:
        NInvState = 40
        MTorqueLimitNegativeFR = -204.1
        MTorqueLimitPositiveFR = 214.2
      (default) -> Encoder_Reset_FR.Inverter_HV_Checks3.Inverter_IN
      (junction 718) -> Encoder_Reset_FR.Inverter_HV_Checks3.Inverter_IN [order 1] : [BInvErrorFR==0]
      Encoder_Reset_FR.Inverter_HV_Checks3.Inv_Error_Check_2 -> (junction 718) : after(500,tick)
      (junction 718) -> Encoder_Reset_FR.Inverter_HV_Checks3.Inv_Error_Check_1 [order 2] : [BInvErrorFR==1]
      Encoder_Reset_FR.Inverter_HV_Checks3.Inv_Error_Reset -> Encoder_Reset_FR.Inverter_HV_Checks3.Inv_Error_Check_2 : after(500,tick)
      Encoder_Reset_FR.Inverter_HV_Checks3.Inverter_IN -> Encoder_Reset_FR.Inverter_HV_Checks3.START_UP : [BInvQuitDcOnFR==1]
      Encoder_Reset_FR.Inverter_HV_Checks3.START_UP -> Encoder_Reset_FR.Inverter_HV_Checks3.Inverter_ON : after(100,tick)
      Encoder_Reset_FR.Inverter_HV_Checks3.Inv_Error_Check_1 -> Encoder_Reset_FR.Inverter_HV_Checks3.Inv_Error_Reset : after(500,tick)
      Encoder_Reset_FR.Inverter_HV_Checks3.Inverter_ON -> Encoder_Reset_FR.Inverter_HV_Checks3.TorqueReq_Ready [order 1] : [BQuitInvOnFR == 1]
      Encoder_Reset_FR.Inverter_HV_Checks3.Inverter_ON -> Encoder_Reset_FR.Inverter_HV_Checks3.Inv_Error_Check_1 [order 2] : [BInvErrorFR==1]
      Encoder_Reset_FR.Inverter_HV_Checks3.TorqueReq_Ready -> Encoder_Reset_FR.Inverter_HV_Checks3.Inv_Error_Check_1 [order 1] : [BInvErrorFR==1]
    state Encoder_OK
      entry:
      NInvState = 41
    (default) -> Encoder_Error_FR
    Encoder_Reset_FR.Encoder_Error_FR.Error_off -> Encoder_Reset_FR.Inverter_HV_Checks3 [order 1] : [BInvSysReadyFR==1]
    Encoder_Reset_FR.Inverter_HV_Checks3.TorqueReq_Ready -> Encoder_Reset_FR.Encoder_OK [order 2] : [BInvErrorFR==0]
  (default) -> Inv_State_Idle
  Inv_State_Idle -> Inv_Error_Checks : [after (4000,tick)]
  Inverter_DCOFF -> Inv_State_Idle : [VDCInvRL<60]
  Inv_OK -> Inverter_DCOFF [order 1] : [VDCInvRL<400]
  Inv_OK -> Inv_Error_Checks [order 2] : [BErrorReset==1]
  Encoder_Reset_RL -> Inv_OK : [NInvState == 26]
  Inv_OK -> Encoder_Reset_RL [order 4] : [NInvDTCRL~=0 && NInvDTCRL~=2359 &&...
      | NInvDTCRL~=1049 && nMotorRL < 5000]
  Inverter_HV_Checks -> Inv_Error_Checks [order 1] : [BErrorReset==1]
  Inv_Error_Checks -> Inverter_HV_Checks : [VDCInvRL>60&&...
      | abs(VHVDelta)<10]
  Encoder_Reset_RR -> Inv_OK : [NInvState == 31]
  Inv_OK -> Encoder_Reset_RR [order 6] : [NInvDTCRR~=0 && NInvDTCRL~=2359 &&...
      | NInvDTCRR~=1049 && nMotorRR < 5000]
  Encoder_Reset_FL -> Inv_OK : [NInvState == 36]
  Inv_OK -> Encoder_Reset_FL [order 5] : [NInvDTCFL~=0 && NInvDTCRL~=2359 &&...
      | NInvDTCFL~=1049 && nMotorFL < 5000]
  Inverter_HV_Checks -> Inv_OK [order 2] : [NInvState==21]
  Encoder_Reset_FR -> Inv_OK : [NInvState == 41]
  Inv_OK -> Encoder_Reset_FR [order 3] : [NInvDTCFR~=0 && NInvDTCRL~=2359 &&...
      | NInvDTCFR~=1049 && nMotorFR < 5000]
  data: NInvState output double; BErrorReset input boolean; VDCInvRL input double; VHVDelta input double; nMotorRL input double; BInvErrorRL input boolean; BInvErrorRR input boolean; BInvErrorFL input boolean; BInvErrorFR input boolean; NInvDTCRL input double; NInvDTCRR input double; NInvDTCFL input double; NInvDTCFR input double; BInvSysReadyRL input boolean; BInvSysReadyRR input boolean; BInvSysReadyFL input boolean; BInvSysReadyFR input boolean; BQuitInvOnRL input boolean; BQuitInvOnRR input boolean; BQuitInvOnFL input boolean; BQuitInvOnFR input boolean; BInvQuitDcOnRL input boolean; BInvQuitDcOnRR input boolean; BHVOn output double; BInvOnRLOut output double; BInvOnRROut output double; BInvOnFLOut output double; BInvOnFROut output double; BInvDCOnRLOut output double; BInvDCOnRROut output double; BInvDCOnFLOut output double; BInvDCOnFROut output double; BInvEnableRL output double; BInvEnableRR output double; BInvEnableFL output double; BInvEnableFR output double; BInvErrorResetRL output double; BInvErrorResetRR output double; BInvErrorResetFL output double; BInvErrorResetFR output double; MTargetTorqueRL output double; MTargetTorqueRR output double; MTargetTorqueFL output double; MTargetTorqueFR output double; MTorqueLimitNegativeRL output double; MTorqueLimitNegativeRR output double; BInvQuitDcOnFL input boolean; MTorqueLimitNegativeFL output double; MTorqueLimitNegativeFR output double; MTorqueLimitPositiveRL output double; MTorqueLimitPositiveRR output double; MTorqueLimitPositiveFL output double; BInvQuitDcOnFR input boolean; MTorqueLimitPositiveFR output double; nMotorRR input double; nMotorFR input double; nMotorFL input double
